simulink model "Plant_inversion_perturbed"  (R2019b)
settings: Solver=ode3  StartTime=-12  StopTime=13  FixedStep=0.001  RelTol=1e-3
settings Model: Creator=Aurelio Piazzi  LastModifiedBy=Aurus

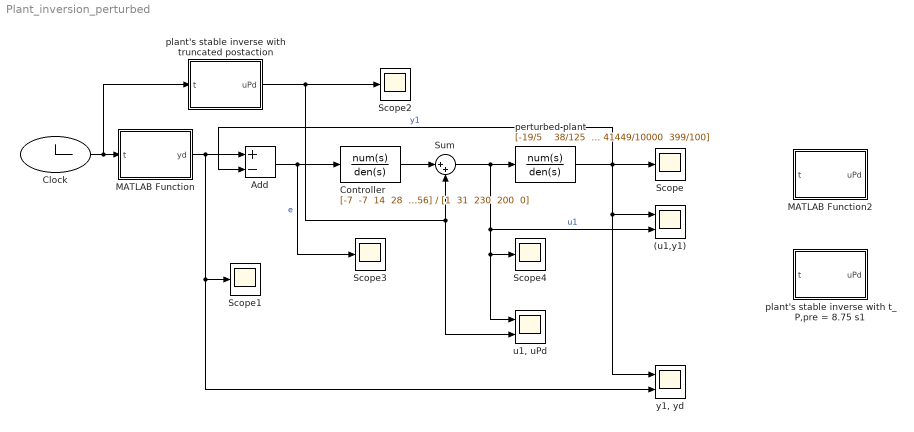
== system Plant_inversion_perturbed ==
  (u1,y1) : Scope  NumInputPorts=2
  Add : Sum  Inputs=+-
  Clock : Clock
  Controller : TransferFcn  Numerator="[-7  -7  14  28  56]"  Denominator="[1  31  230  200  0]"
  MATLAB Function : MATLAB Function  TreatAsAtomicUnit=on
  MATLAB Function2 : MATLAB Function  TreatAsAtomicUnit=on
  Scope{,1..4} (5 alike) : Scope
  Sum : Sum  Inputs=|++
  perturbed plant : TransferFcn  Numerator="[-19/5    38/125   38703/10000]"  Denominator="[1/100    2063/2000  63821/20000   41449/10000  399/100]"
  plant's stable inverse with t_P,pre = 8.75 s1 : MATLAB Function  TreatAsAtomicUnit=on
  plant's stable inverse with truncated postaction : MATLAB Function  TreatAsAtomicUnit=on
  "u1, uPd" : Scope  NumInputPorts=2
  "y1, yd" : Scope  NumInputPorts=2
  wires:
  MATLAB Function/1(yd) -> "y1, yd"/2, Scope1/1, Add/1
  Add/1 -> Controller/1, Scope3/1  "e"
  perturbed plant/1 -> (u1,y1)/1, "y1, yd"/1, Scope/1, Add/2  "y1"
  Clock/1 -> plant's stable inverse with truncated postaction/1(t), MATLAB Function/1(t)
  Controller/1 -> Sum/1
  Sum/1 -> (u1,y1)/2, "u1, uPd"/1, Scope4/1, perturbed plant/1  "u1"
  plant's stable inverse with truncated postaction/1(uPd) -> Scope2/1, "u1, uPd"/2, Sum/2

== matlab function Plant_inversion_perturbed/plant's stable inverse with truncated postaction ==
  data: t input; uPd output
function uPd = uPd(t)
 if(t<0)
     uPd = (1/3)*exp(t)+(5/3)*exp(t-3);
 elseif (t<3)
     uPd = -(1/9)*t+(1/9)*t^2-(2/27)*t^3-(5/18)*exp(-t)+11/18+(5/3)*exp(t-3);
 elseif (t < 3 + 6.96)
     uPd = 1-(5/18)*exp(-t)-(1/18)*exp(3-t);
 else
     uPd = 1;
 end

== matlab function Plant_inversion_perturbed/MATLAB Function ==
  data: t input; yd output
function yd = yd(t)
 if(t<0)
     yd = 0;
 elseif (t<3)
     yd = (1/3)*t^2-(2/27)*t^3;
 else
     yd = 1;
 end

== matlab function Plant_inversion_perturbed/MATLAB Function2 ==
  data: t input; uPd output
function uPd = uPd(t)
 if(t<0)
     uPd = (1/3)*exp(t)+(5/3)*exp(t-3);
 elseif (t<3)
     uPd = -(1/9)*t+(1/9)*t^2-(2/27)*t^3-(5/18)*exp(-t)+11/18+(5/3)*exp(t-3);
 else
     uPd = 1-(5/18)*exp(-t)-(1/18)*exp(3-t);
 end

== matlab function Plant_inversion_perturbed/plant's stable inverse with t_P,pre = 8.75 s1 ==
  data: t input; uPd output
function uPd = uPd(t)
 if (t<-8.75)
     uPd = 0;
 elseif(t<0)
     uPd = (1/3)*exp(t)+(5/3)*exp(t-3);
 elseif (t<3)
     uPd = -(1/9)*t+(1/9)*t^2-(2/27)*t^3-(5/18)*exp(-t)+11/18+(5/3)*exp(t-3);
 else
     uPd = 1-(5/18)*exp(-t)-(1/18)*exp(3-t);
 end
